simulink model "PMSM_Drive_Controller"  (R2018a)
settings: Solver=VariableStepDiscrete  StartTime=0.0  StopTime=15  RelTol=1e-3
libraries: powerlib x24, simulink x3, powerlib_meascontrol x1
settings Model: Creator=bulbu  LastModifiedBy=bulbu
settings SolverCC: ZeroCrossAlgorithm=Adaptive
settings DebuggingCC: MaxConsecutiveZCsMsg=none  IgnoredZcDiagnostic=none

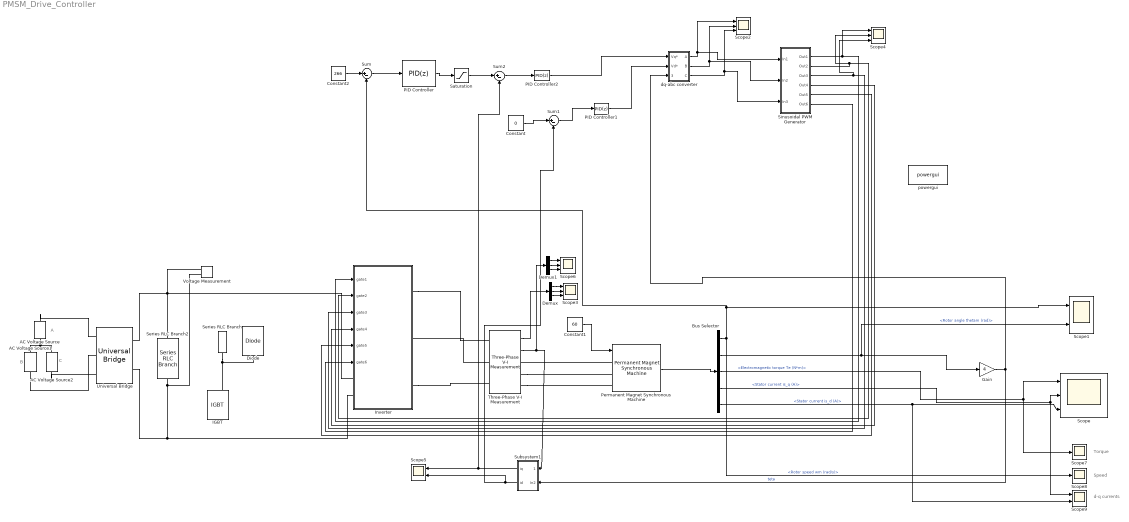
== system PMSM_Drive_Controller ==
  note: A
  note: Torque
  note: Speed
  note: d-q currents
  note: C
  note: B
  AC Voltage Source : powerlib/Electrical Sources/AC Voltage Source  Amplitude=326.6  Phase=0  Frequency=50  SampleTime=0  Measurements=None  BusType=swing  Pref=10e3  Qref=0  Qmin=-inf  Qmax=+inf
  AC Voltage Source1 : powerlib/Electrical Sources/AC Voltage Source  Amplitude=326.6  Phase=120  Frequency=50  SampleTime=0  Measurements=None  BusType=swing  Pref=10e3  Qref=0  Qmin=-inf  Qmax=+inf
  AC Voltage Source2 : powerlib/Electrical Sources/AC Voltage Source  Amplitude=326.6  Phase=240  Frequency=50  SampleTime=0  Measurements=None  BusType=swing  Pref=10e3  Qref=0  Qmin=-inf  Qmax=+inf
  Bus Selector : BusSelector  OutputSignals=Rotor speed wm (rad/s),Rotor angle thetam (rad),Electromagnetic torque Te (N*m),Stator current is_q (A),Stator current is_d (A)
  Constant : Constant  Value=0
  Constant1 : Constant  Value=60
  Constant2 : Constant  Value=266
  Demux : Demux  Outputs=3
  Demux1 : Demux  Outputs=3
  Diode : powerlib/Power Electronics/Diode  Ron=0.001  Lon=0  Vf=0.8  IC=0  UseSnubber=0  Rs=500  Cs=250e-9  Measurements=off
  Gain : Gain  Gain=4
  IGBT : powerlib/Power Electronics/IGBT  Ron=0.001  Lon=0  Vf=1  Tf=1e-6  Tt=2e-6  IC=0  Rs=1e5  Cs=inf  Measurements=off
  "Inverter " : Subsystem
  PID Controller : simulink/Continuous/PID Controller  Controller=PID  TimeDomain=Discrete-time  SampleTime=-1  IntegratorMethod=Forward Euler  FilterMethod=Forward Euler  Form=Parallel  UseFilter=on  ControllerParametersSource=internal  P=990  I=6  D=0  N=100  InitialConditionSource=internal  InitialConditionForIntegrator=0  InitialConditionForFilter=0  ExternalReset=none  LimitOutput=off  UpperSaturationLimit=inf  LowerSaturationLimit=-inf  LinearizeAsGain=on  AntiWindupMode=none  Kb=1  TrackingMode=off  Kt=1  PParamMin=[]  PParamMax=[]  IParamMin=[]  IParamMax=[]  DParamMin=[]  DParamMax=[]  NParamMin=[]  NParamMax=[]  KbParamMin=[]  KbParamMax=[]  KtParamMin=[]  KtParamMax=[]  POutMin=[]  POutMax=[]  IOutMin=[]  IOutMax=[]  DOutMin=[]  DOutMax=[]  NOutMin=[]  NOutMax=[]  KbOutMin=[]  KbOutMax=[]  KtOutMin=[]  KtOutMax=[]  IntegratorOutMin=[]  IntegratorOutMax=[]  FilterOutMin=[]  FilterOutMax=[]  SumOutMin=[]  SumOutMax=[]  SumI1OutMin=[]  SumI1OutMax=[]  SumI2OutMin=[]  SumI2OutMax=[]  SumI3OutMin=[]  SumI3OutMax=[]  SumDOutMin=[]  SumDOutMax=[]  SaturationOutMin=[]  SaturationOutMax=[]  IntegratorContinuousStateAttributes=''  IntegratorStateMustResolveToSignalObject=off  IntegratorRTWStateStorageClass=Auto  FilterContinuousStateAttributes=''  FilterStateMustResolveToSignalObject=off  FilterRTWStateStorageClass=Auto  DifferentiatorICPrevScaledInput=0  DifferentiatorOutMin=[]  DifferentiatorOutMax=[]  FilterDiffOutCoefMin=[]  FilterDiffOutCoefMax=[]  SumDenOutMin=[]  SumDenOutMax=[]  SumNumOutMin=[]  SumNumOutMax=[]  ReciprocalOutMin=[]  ReciprocalOutMax=[]  DivideOutMin=[]  DivideOutMax=[]  TunerSelectOption=Transfer Function Based (PID Tuner App)
  PID Controller1 : simulink/Continuous/PID Controller  Controller=PID  TimeDomain=Discrete-time  SampleTime=-1  IntegratorMethod=Forward Euler  FilterMethod=Forward Euler  Form=Parallel  UseFilter=on  ControllerParametersSource=internal  P=0.01  I=1000  D=10  N=100  InitialConditionSource=internal  InitialConditionForIntegrator=0  InitialConditionForFilter=0  ExternalReset=none  LimitOutput=off  UpperSaturationLimit=inf  LowerSaturationLimit=-inf  LinearizeAsGain=on  AntiWindupMode=none  Kb=1  TrackingMode=off  Kt=1  PParamMin=[]  PParamMax=[]  IParamMin=[]  IParamMax=[]  DParamMin=[]  DParamMax=[]  NParamMin=[]  NParamMax=[]  KbParamMin=[]  KbParamMax=[]  KtParamMin=[]  KtParamMax=[]  POutMin=[]  POutMax=[]  IOutMin=[]  IOutMax=[]  DOutMin=[]  DOutMax=[]  NOutMin=[]  NOutMax=[]  KbOutMin=[]  KbOutMax=[]  KtOutMin=[]  KtOutMax=[]  IntegratorOutMin=[]  IntegratorOutMax=[]  FilterOutMin=[]  FilterOutMax=[]  SumOutMin=[]  SumOutMax=[]  SumI1OutMin=[]  SumI1OutMax=[]  SumI2OutMin=[]  SumI2OutMax=[]  SumI3OutMin=[]  SumI3OutMax=[]  SumDOutMin=[]  SumDOutMax=[]  SaturationOutMin=[]  SaturationOutMax=[]  IntegratorContinuousStateAttributes=''  IntegratorStateMustResolveToSignalObject=off  IntegratorRTWStateStorageClass=Auto  FilterContinuousStateAttributes=''  FilterStateMustResolveToSignalObject=off  FilterRTWStateStorageClass=Auto  DifferentiatorICPrevScaledInput=0  DifferentiatorOutMin=[]  DifferentiatorOutMax=[]  FilterDiffOutCoefMin=[]  FilterDiffOutCoefMax=[]  SumDenOutMin=[]  SumDenOutMax=[]  SumNumOutMin=[]  SumNumOutMax=[]  ReciprocalOutMin=[]  ReciprocalOutMax=[]  DivideOutMin=[]  DivideOutMax=[]  TunerSelectOption=Transfer Function Based (PID Tuner App)
  PID Controller2 : simulink/Continuous/PID Controller  Controller=PID  TimeDomain=Discrete-time  SampleTime=-1  IntegratorMethod=Forward Euler  FilterMethod=Forward Euler  Form=Parallel  UseFilter=on  ControllerParametersSource=internal  P=0.01  I=1000  D=2  N=100  InitialConditionSource=internal  InitialConditionForIntegrator=0  InitialConditionForFilter=0  ExternalReset=none  LimitOutput=off  UpperSaturationLimit=inf  LowerSaturationLimit=-inf  LinearizeAsGain=on  AntiWindupMode=none  Kb=1  TrackingMode=off  Kt=1  PParamMin=[]  PParamMax=[]  IParamMin=[]  IParamMax=[]  DParamMin=[]  DParamMax=[]  NParamMin=[]  NParamMax=[]  KbParamMin=[]  KbParamMax=[]  KtParamMin=[]  KtParamMax=[]  POutMin=[]  POutMax=[]  IOutMin=[]  IOutMax=[]  DOutMin=[]  DOutMax=[]  NOutMin=[]  NOutMax=[]  KbOutMin=[]  KbOutMax=[]  KtOutMin=[]  KtOutMax=[]  IntegratorOutMin=[]  IntegratorOutMax=[]  FilterOutMin=[]  FilterOutMax=[]  SumOutMin=[]  SumOutMax=[]  SumI1OutMin=[]  SumI1OutMax=[]  SumI2OutMin=[]  SumI2OutMax=[]  SumI3OutMin=[]  SumI3OutMax=[]  SumDOutMin=[]  SumDOutMax=[]  SaturationOutMin=[]  SaturationOutMax=[]  IntegratorContinuousStateAttributes=''  IntegratorStateMustResolveToSignalObject=off  IntegratorRTWStateStorageClass=Auto  FilterContinuousStateAttributes=''  FilterStateMustResolveToSignalObject=off  FilterRTWStateStorageClass=Auto  DifferentiatorICPrevScaledInput=0  DifferentiatorOutMin=[]  DifferentiatorOutMax=[]  FilterDiffOutCoefMin=[]  FilterDiffOutCoefMax=[]  SumDenOutMin=[]  SumDenOutMax=[]  SumNumOutMin=[]  SumNumOutMax=[]  ReciprocalOutMin=[]  ReciprocalOutMax=[]  DivideOutMin=[]  DivideOutMax=[]  TunerSelectOption=Transfer Function Based (PID Tuner App)
  Permanent Magnet Synchronous Machine : powerlib/Machines/Permanent Magnet Synchronous Machine  NbPhases=3  FluxDistribution=Sinusoidal  RotorType=Round  MechanicalLoad=Torque Tm  PresetModel=No  ShowDetailedParameters=on  MeasurementBus=off  Resistance=50e-3  Inductance=8.5e-3  dqInductances=[500e-6,500e-6]  La=500e-6  MachineConstant=Flux linkage established by magnets (V.s)  Flux=0.2  VoltageCst=145.1039  TorqueCst=1.2  Flat=120  Mechanical=[10 0 4 0]  PolePairs=4  InitialConditions=[0,0, 0,0]  InitialConditions5ph=[0 0 0 0 0 0]  TsPowergui=0  TsBlock=-1  RefAngle=90 degrees behind phase A axis (modified Park)
      settings: SourceProductName=Simscape Power Systems
  Saturation : Saturate  UpperLimit=250  LowerLimit=-250
  Scope{,2..4,6} (5 alike) : Scope  NumInputPorts=3
  Scope1 : Scope  NumInputPorts=2
  Scope5 : Scope  NumInputPorts=2
  Scope7 : Scope
  Scope8 : Scope
  Scope9 : Scope  NumInputPorts=2
  Series RLC Branch : powerlib/Elements/Series RLC Branch  LConnTagsString=__new0  RConnTagsString=__new0  BranchType=R  Resistance=1  Inductance=1e-3  SetiL0=off  InitialCurrent=0  Capacitance=1e-6  Setx0=off  InitialVoltage=0  Measurements=None
  Series RLC Branch2 : powerlib/Elements/Series RLC Branch  LConnTagsString=__new0  RConnTagsString=__new0  BranchType=C  Resistance=2.16  Inductance=1e-3  SetiL0=off  InitialCurrent=0  Capacitance=990e-6  Setx0=off  InitialVoltage=0  Measurements=None
  "Sinusoidal PWM Generator " : Subsystem
  Subsystem1 : Subsystem
  Sum : Sum  Inputs=|+-
  Sum1 : Sum  Inputs=|+-
  Sum2 : Sum  Inputs=|+-
  Three-Phase V-I Measurement : powerlib/Measurements/Three-Phase V-I Measurement  VoltageMeasurement=phase-to-phase  SetLabelV=off  LabelV=Vabc  Vpu=off  VpuLL=off  CurrentMeasurement=yes  SetLabelI=off  LabelI=Iabc  Ipu=off  Pbase=100e6  Vbase=500e3  OutputType=Complex  PhasorSimulation=off  PSBequivalent=0
  Universal Bridge : powerlib/Power Electronics/Universal Bridge  Arms=3  SnubberResistance=1e5  SnubberCapacitance=inf  Device=Diodes  Ron=1e-3  Lon=0  ForwardVoltages="[  0  0  ]"  ForwardVoltage=0  GTOparameters=[ 10e-6 , 20e-6 ]  IGBTparameters=[ 1e-6 , 2e-6 ]  Measurements=None  Measurements_2=None  converterType=Rectifier
  Voltage Measurement : powerlib/Measurements/Voltage Measurement  PhasorSimulation=off  OutputType=Complex  PSBequivalent=0
  "dq-abc converter " : Subsystem
  powergui : powerlib/powergui  Priority=1  SimulationMode=Discrete  SampleTime=1e-5  frequency=60  Iterations=50  frequencyindice=0  Pbase=100e6  ErrMax=1e-4  UnitsV=kV  UnitsW=MW  buscounter=0  FunctionMessages=off  echomessages=off  EnableUseOfTLC=off  CurrentSourceSwitches=off  DisableSnubberDevices=off  DisableRonSwitches=off  DisableVfSwitches=off  DisplayEquations=off  SolverType=Tustin/Backward Euler (TBE)  Interpol=off  ExternalGateDelay=off  methode=off  Ts=100  x0status=blocks  SPID=on  SwTol=0  HookPort=off  RestoreLinks=warning  ResistiveCurrentMeasurement=off  Frange=[0:2:500]  Ylog=off  Xlog=on  ShowGrid=off  save=off  variable=ZData  structure=0  ZoomFFT=off  StartTime=0.0  cycles=1  DisplayStyle=1  fundamental=60  FreqAxis=off  MaxFrequency=1000  frequencyindicesteady=1  RmsSteady=1  display=off
  wires:
  Sum/1 -> PID Controller/1
  Permanent Magnet Synchronous Machine/1 -> Bus Selector/1
  Bus Selector/2 -> Scope1/2, Gain/1  "<Rotor angle thetam (rad)>"
  Bus Selector/3 -> Scope7/1, Scope/1  "<Electromagnetic torque Te (N*m)>"
  Bus Selector/4 -> Scope9/1, Scope/2  "<Stator current is_q (A)>"
  Bus Selector/5 -> Scope9/2, Scope/3  "<Stator current is_d (A)>"
  Constant2/1 -> Sum/1
  "dq-abc converter "/1(A) -> Scope2/1, "Sinusoidal PWM Generator "/1(In1)
  "dq-abc converter "/2(B) -> Scope2/2, "Sinusoidal PWM Generator "/2(In2)
  "dq-abc converter "/3(C) -> Scope2/3, "Sinusoidal PWM Generator "/3(In3)
  "Sinusoidal PWM Generator "/1(Out1) -> Scope4/1, "Inverter "/1(gate1)
  "Sinusoidal PWM Generator "/2(Out2) -> Scope4/2, "Inverter "/2(gate2)
  "Sinusoidal PWM Generator "/3(Out3) -> Scope4/3, "Inverter "/3(gate3)
  "Sinusoidal PWM Generator "/4(Out4) -> "Inverter "/4(gate4)
  "Sinusoidal PWM Generator "/5(Out5) -> "Inverter "/5(gate5)
  "Sinusoidal PWM Generator "/6(Out6) -> "Inverter "/6(gate6)
  Gain/1 -> Subsystem1/2(In2), "dq-abc converter "/3("teta ")  "teta"
  Sum1/1 -> PID Controller1/1
  Constant/1 -> Sum1/1
  Sum2/1 -> PID Controller2/1
  Three-Phase V-I Measurement/2 -> Demux1/1, Subsystem1/1("iabc ")
  PID Controller/1 -> Saturation/1
  Saturation/1 -> Sum2/1
  Subsystem1/2(id) -> Scope5/2, Sum1/2
  Subsystem1/1(iq) -> Scope5/1, Sum2/2
  Bus Selector/1 -> Scope8/1, Sum/2, Scope1/1  "<Rotor speed wm (rad/s)>"
  PID Controller2/1 -> "dq-abc converter "/1(Vq*)
  PID Controller1/1 -> "dq-abc converter "/2(Vd*)
  Constant1/1 -> Permanent Magnet Synchronous Machine/1
  Three-Phase V-I Measurement/1 -> Demux/1
  Demux/3 -> Scope3/3
  Demux/1 -> Scope3/1
  Demux/2 -> Scope3/2
  Demux1/3 -> Scope6/3
  Demux1/1 -> Scope6/1
  Demux1/2 -> Scope6/2
  connections:
  Permanent Magnet Synchronous Machine/LConn1 -- Three-Phase V-I Measurement/RConn1
  Three-Phase V-I Measurement/RConn2 -- Permanent Magnet Synchronous Machine/LConn2
  Three-Phase V-I Measurement/RConn3 -- Permanent Magnet Synchronous Machine/LConn3
  Universal Bridge/RConn2 -- "Inverter "/LConn2 -- Voltage Measurement/LConn2 -- Series RLC Branch2/RConn1
  Series RLC Branch2/LConn1 -- Universal Bridge/RConn1 -- "Inverter "/LConn1 -- Voltage Measurement/LConn1
  AC Voltage Source/LConn1 -- AC Voltage Source2/LConn1 -- AC Voltage Source1/LConn1
  AC Voltage Source/RConn1 -- Universal Bridge/LConn1
  AC Voltage Source2/RConn1 -- Universal Bridge/LConn3
  AC Voltage Source1/RConn1 -- Universal Bridge/LConn2
  "Inverter "/RConn1 -- Three-Phase V-I Measurement/LConn1
  Three-Phase V-I Measurement/LConn2 -- "Inverter "/RConn2
  "Inverter "/RConn3 -- Three-Phase V-I Measurement/LConn3
  Series RLC Branch/RConn1 -- Diode/LConn1 -- IGBT/LConn1

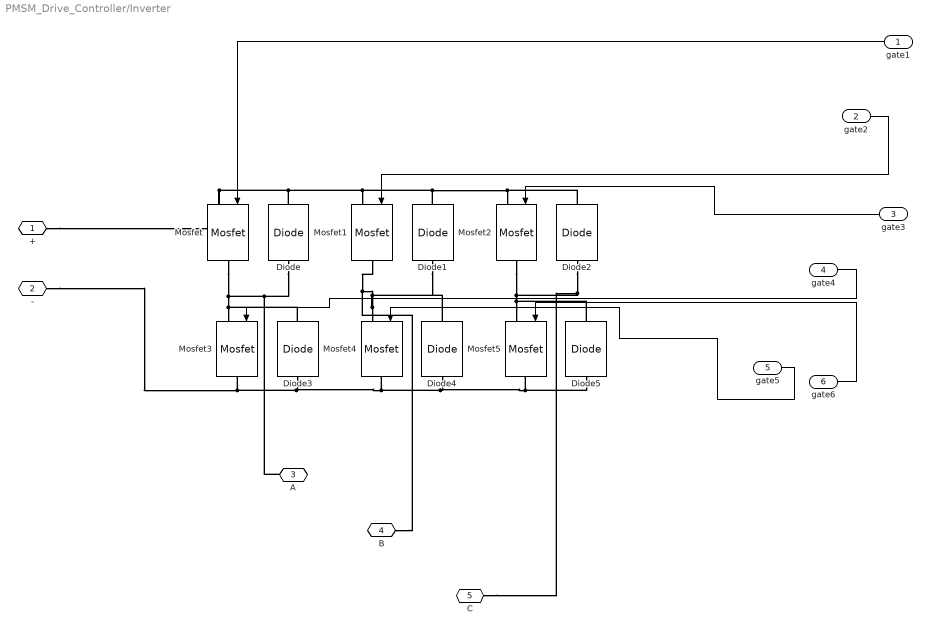
== system PMSM_Drive_Controller/Inverter  ==
  gate1 : Inport
  gate2 : Inport  Port=2
  gate3 : Inport  Port=3
  gate4 : Inport  Port=4
  gate5 : Inport  Port=5
  gate6 : Inport  Port=6
  Diode{,1..5} (6 alike) : powerlib/Power Electronics/Diode  Ron=0.001  Lon=0  Vf=0.8  IC=0  UseSnubber=0  Rs=500  Cs=250e-9  Measurements=off
  Mosfet{,1..5} (6 alike) : powerlib/Power Electronics/Mosfet  Ron=0.1  Lon=0  Rd=0.01  Vfd=0  IC=0  Rs=1e5  Cs=inf  Measurements=off
  + : PMIOPort  Side=Left
  - : PMIOPort  Port=2  Side=Left
  A : PMIOPort  Port=3  Side=Right
  B : PMIOPort  Port=4  Side=Right
  C : PMIOPort  Port=5  Side=Right
  wires:
  gate3/1 -> Mosfet2/1
  gate4/1 -> Mosfet3/1
  gate2/1 -> Mosfet1/1
  gate5/1 -> Mosfet4/1
  gate6/1 -> Mosfet5/1
  gate1/1 -> Mosfet/1
  connections:
  Diode5/LConn1 -- Diode3/LConn1 -- -/RConn1 -- Mosfet3/RConn1 -- Mosfet4/RConn1 -- Diode4/LConn1 -- Mosfet5/RConn1
  Diode1/LConn1 -- B/RConn1 -- Mosfet1/RConn1 -- Diode4/RConn1 -- Mosfet4/LConn1
  Mosfet5/LConn1 -- Mosfet2/RConn1 -- C/RConn1 -- Diode2/LConn1 -- Diode5/RConn1
  Mosfet/LConn1 -- +/RConn1 -- Mosfet2/LConn1 -- Diode2/RConn1 -- Diode1/RConn1 -- Mosfet1/LConn1 -- Diode/RConn1
  Mosfet/RConn1 -- Diode3/RConn1 -- Mosfet3/LConn1 -- A/RConn1 -- Diode/LConn1

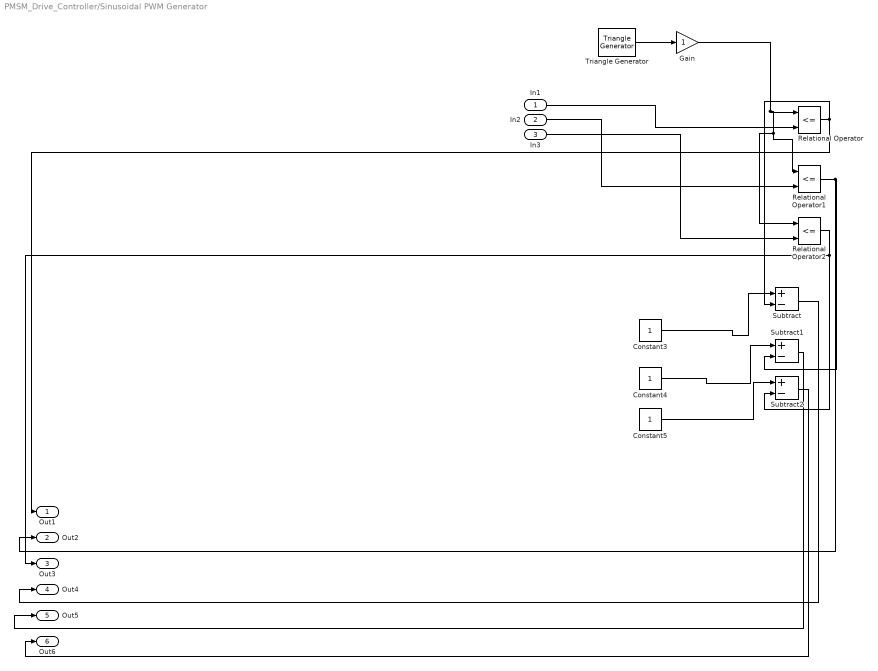
== system PMSM_Drive_Controller/Sinusoidal PWM Generator  ==
  In1 : Inport
  In2 : Inport  Port=2
  In3 : Inport  Port=3
  Constant3 : Constant
  Constant4 : Constant
  Constant5 : Constant
  Gain : Gain
  Relational Operator : RelationalOperator  Operator=<=  OutDataTypeStr=boolean  RndMeth=Simplest
  Relational Operator1 : RelationalOperator  Operator=<=  OutDataTypeStr=boolean  RndMeth=Simplest
  Relational Operator2 : RelationalOperator  Operator=<=  OutDataTypeStr=boolean  RndMeth=Simplest
  Subtract : Sum  Inputs=+-
  Subtract1 : Sum  Inputs=+-
  Subtract2 : Sum  Inputs=+-
  Triangle Generator : powerlib_meascontrol/Pulse & Signal Generators/Triangle Generator  Freq=20000  Phase=90  Ts=0
  Out1 : Outport
  Out2 : Outport  Port=2
  Out3 : Outport  Port=3
  Out4 : Outport  Port=4
  Out5 : Outport  Port=5
  Out6 : Outport  Port=6
  wires:
  Subtract2/1 -> Out6/1
  Relational Operator/1 -> Out1/1, Subtract/2
  Constant5/1 -> Subtract2/1
  Relational Operator2/1 -> Out3/1, Subtract2/2
  Subtract1/1 -> Out5/1
  Constant4/1 -> Subtract1/1
  Relational Operator1/1 -> Out2/1, Subtract1/2
  Triangle Generator/1 -> Gain/1
  Constant3/1 -> Subtract/1
  Subtract/1 -> Out4/1
  In1/1 -> Relational Operator/2
  In3/1 -> Relational Operator2/2
  In2/1 -> Relational Operator1/2
  Gain/1 -> Relational Operator2/1, Relational Operator1/1, Relational Operator/1

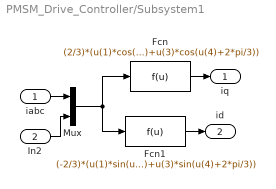
== system PMSM_Drive_Controller/Subsystem1 ==
  "iabc " : Inport
  In2 : Inport  Port=2
  Fcn : Fcn  Expr=(2/3)*(u(1)*cos(u(4))+u(2)*cos(u(4)-2*pi/3)+u(3)*cos(u(4)+2*pi/3))
  Fcn1 : Fcn  Expr=(-2/3)*(u(1)*sin(u(4))+u(2)*sin(u(4)-2*pi/3)+u(3)*sin(u(4)+2*pi/3))
  Mux : Mux  Inputs=2
  iq : Outport
  id : Outport  Port=2
  wires:
  In2/1 -> Mux/2
  Mux/1 -> Fcn1/1, Fcn/1
  Fcn1/1 -> id/1
  Fcn/1 -> iq/1
  "iabc "/1 -> Mux/1

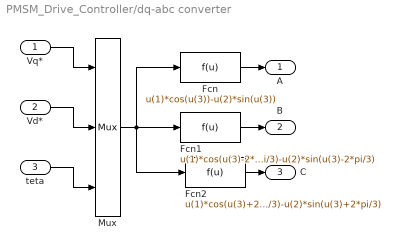
== system PMSM_Drive_Controller/dq-abc converter  ==
  Vq* : Inport
  Vd* : Inport  Port=2
  "teta " : Inport  Port=3
  Fcn : Fcn  Expr=u(1)*cos(u(3))-u(2)*sin(u(3))
  Fcn1 : Fcn  Expr=u(1)*cos(u(3)-2*pi/3)-u(2)*sin(u(3)-2*pi/3)
  Fcn2 : Fcn  Expr=u(1)*cos(u(3)+2*pi/3)-u(2)*sin(u(3)+2*pi/3)
  Mux : Mux  Inputs=3
  A : Outport
  B : Outport  Port=2
  C : Outport  Port=3
  wires:
  Mux/1 -> Fcn/1, Fcn2/1, Fcn1/1
  Fcn/1 -> A/1
  "teta "/1 -> Mux/3
  Vd*/1 -> Mux/2
  Vq*/1 -> Mux/1
  Fcn1/1 -> B/1
  Fcn2/1 -> C/1
